simulink model "be503_miniProject"  (R2021a)
settings: Solver=VariableStepAuto  StartTime=0.0  StopTime=3  RelTol=1e-3
values from neighbouring files (symbols this model uses):
  den_high = den_high{1}    [record.m]
  den_low_pass = den_low_pass{1}    [record.m]
  myRecording = getaudiodata(z)    [record.m]
  num_high = num_high{1}    [record.m]
  num_low_pass = num_low_pass{1}    [record.m]
libraries: simulink x1
settings Model: Creator=pongthang  LastModifiedBy=pongthang

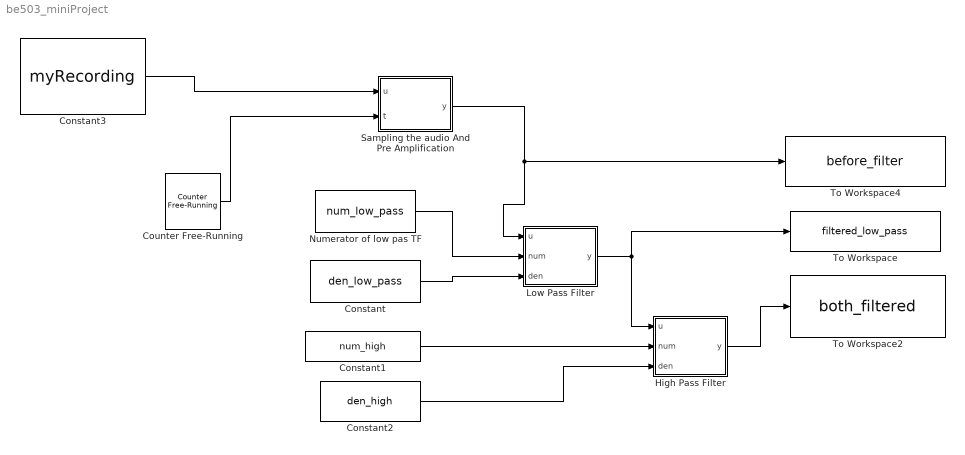
== system be503_miniProject ==
  Constant : Constant  Value=den_low_pass
  Constant1 : Constant  Value=num_high
  Constant2 : Constant  Value=den_high
  Constant3 : Constant  Value=myRecording
  Counter Free-Running : simulink/Sources/Counter Free-Running  NumBits=16  tsamp=0.000125
  High Pass Filter : MATLAB Function  TreatAsAtomicUnit=on
  Low Pass Filter : MATLAB Function  TreatAsAtomicUnit=on
  Numerator of low pas TF : Constant  Value=num_low_pass
  Sampling the audio And Pre Amplification : MATLAB Function  TreatAsAtomicUnit=on
  To Workspace : ToWorkspace  VariableName=filtered_low_pass  SaveFormat=Timeseries  SampleTime=-1
  To Workspace2 : ToWorkspace  VariableName=both_filtered  SaveFormat=Timeseries  SampleTime=-1
  To Workspace4 : ToWorkspace  VariableName=before_filter  SaveFormat=Timeseries  SampleTime=-1
  wires:
  Low Pass Filter/1(y) -> High Pass Filter/1(u), To Workspace/1
  Numerator of low pas TF/1 -> Low Pass Filter/2(num)
  Constant/1 -> Low Pass Filter/3(den)
  Constant1/1 -> High Pass Filter/2(num)
  Constant2/1 -> High Pass Filter/3(den)
  High Pass Filter/1(y) -> To Workspace2/1
  Counter Free-Running/1 -> Sampling the audio And Pre Amplification/2(t)
  Sampling the audio And Pre Amplification/1(y) -> Low Pass Filter/1(u), To Workspace4/1
  Constant3/1 -> Sampling the audio And Pre Amplification/1(u)

== matlab function be503_miniProject/High Pass Filter ==
  settings: updateMethod=DISCRETE
  data: u input; y output; num input; den input

function y= fcn(u,num,den)
persistent x_1 y_1
if isempty(x_1) 
    x_1=0;
end
if isempty(y_1) 
    y_1=0;
end

y = num(1)*u+num(2)*x_1-den(2)*y_1;
x_1=u;
y_1 = y;
end

== matlab function be503_miniProject/Low Pass Filter ==
  settings: updateMethod=DISCRETE
  data: u input; y output; num input; den input

function y= fcn(u,num,den)
persistent x_1 y_1
if isempty(x_1) 
    x_1=0;
end
if isempty(y_1) 
    y_1=0;
end

y = num(1)*u+num(2)*x_1-den(2)*y_1;
x_1=u;
y_1 = y;
end

== matlab function be503_miniProject/Sampling the audio And Pre Amplification ==
  data: u input; t input; y output
function y = fcn(u,t)
 if t>0
    y = u(t);
 else
     y=0;
 end
 
end
%35 to 85
